simulink model "observer_tuning"  (R2016b)
settings: Solver=VariableStepAuto  StartTime=0.0  StopTime=10.0  RelTol=1e-3
values from neighbouring files (symbols this model uses):
  A = [0      1              0           0 ... (first row only)    [ImportStateSpace.m]    (also in multi_plot_tune_observer.m = sys.A; multi_plot_tune_observer2.m = sys.A; responseObserver.m = sys.A)
  B = [     0 ... (first row only)    [ImportStateSpace.m]    (also in multi_plot_tune_observer.m = sys.B; multi_plot_tune_observer2.m = sys.B; responseObserver.m = sys.B)
  C = [1 0 0 0 ... (first row only)    [ImportStateSpace.m]    (also in multi_plot_tune_observer.m = sys.C; multi_plot_tune_observer2.m = sys.C; responseObserver.m = sys.C)
  D = zeros(size(C,1), size(B,2))    [ImportStateSpace.m]    (also in multi_plot_tune_observer.m = sys.D; multi_plot_tune_observer2.m = sys.D; responseObserver.m = sys.D)
  K = place(sys.A, sys.B, eigs)    [LCSproject.m]    (also in myLQR.m = lqr(sys.A, sys.B, Q, R))
  kr = -1/(C*inv(A-B*K)*B)    [LCSproject.m]
  L_tuning = place(A',C',Poles)'    [multi_plot_tune_simulink_observer.m]
  simin_delay = 0.001    [multi_plot_tune_simulink_observer.m]
settings Model: Creator=Olivier  LastModifiedBy=Olivier

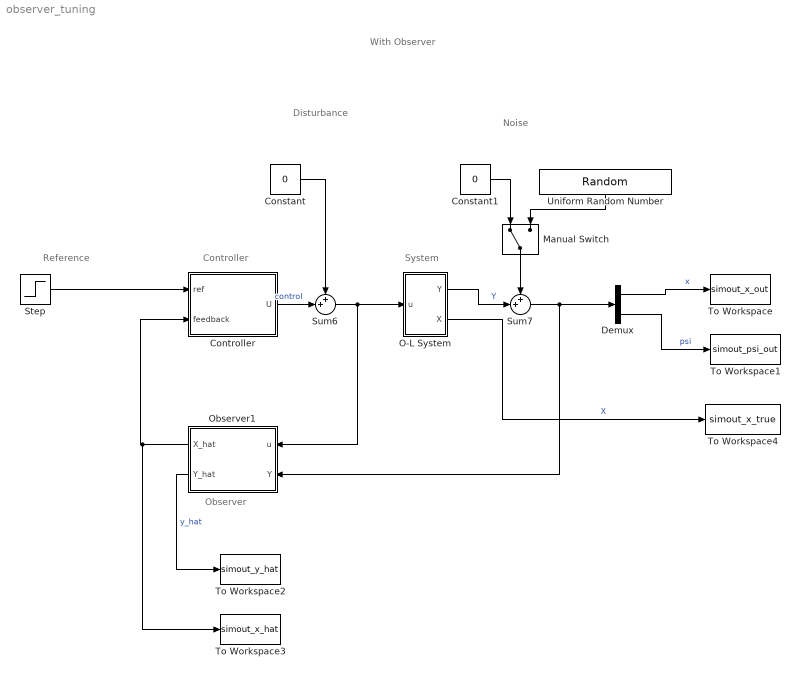
== system observer_tuning ==
  note: With Observer
  note: System
  note: Observer
  note: Controller
  note: Reference
  note: Disturbance
  note: Noise
  Constant : Constant  Value=0
  Constant1 : Constant  Value=0
  Controller : Subsystem
  Demux : Demux  Outputs=2
  Manual Switch : ManualSwitch
  O-L System : Subsystem
  Observer1 : Subsystem
  Step : Step  After=0.2  SampleTime=0
  Sum6 : Sum  Inputs=++|
  Sum7 : Sum  Inputs=++|
  To Workspace : ToWorkspace  VariableName=simout_x_out  SaveFormat=Timeseries  SampleTime=-1
  To Workspace1 : ToWorkspace  VariableName=simout_psi_out  SaveFormat=Timeseries  SampleTime=-1
  To Workspace2 : ToWorkspace  VariableName=simout_y_hat  SaveFormat=Timeseries  SampleTime=-1
  To Workspace3 : ToWorkspace  VariableName=simout_x_hat  SaveFormat=Timeseries  SampleTime=-1
  To Workspace4 : ToWorkspace  VariableName=simout_x_true  SaveFormat=Timeseries  SampleTime=-1
  Uniform Random Number : UniformRandomNumber  Minimum=-0.0001  Maximum=0.0001  SampleTime=0.1
  wires:
  Sum7/1 -> Demux/1, Observer1/2(Y)
  Controller/1(U) -> Sum6/2  "control"
  Observer1/1(X_hat) -> To Workspace3/1, Controller/2(feedback)
  Sum6/1 -> Observer1/1(u), O-L System/1(u)
  Manual Switch/1 -> Sum7/1
  Demux/2 -> To Workspace1/1  "psi"
  Demux/1 -> To Workspace/1  "x"
  O-L System/1(Y) -> Sum7/2  "Y"
  Step/1 -> Controller/1(ref)
  Observer1/2(Y_hat) -> To Workspace2/1  "y_hat"
  O-L System/2(X) -> To Workspace4/1  "X"
  Constant/1 -> Sum6/1
  Uniform Random Number/1 -> Manual Switch/2
  Constant1/1 -> Manual Switch/1

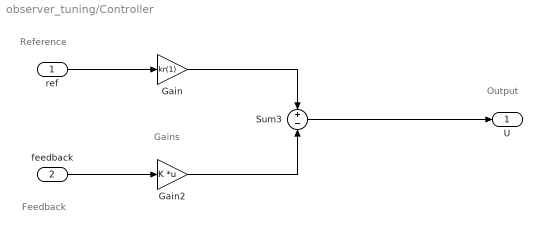
== system observer_tuning/Controller ==
  note: Output
  note: Gains
  note: Feedback
  note: Reference
  ref : Inport
  feedback : Inport  Port=2
  Gain : Gain  Gain=kr(1)
  Gain2 : Gain  Gain=K  Multiplication=Matrix(K*u)
  Sum3 : Sum  Inputs=+|-
  U : Outport
  wires:
  Sum3/1 -> U/1
  Gain2/1 -> Sum3/2
  feedback/1 -> Gain2/1
  ref/1 -> Gain/1
  Gain/1 -> Sum3/1

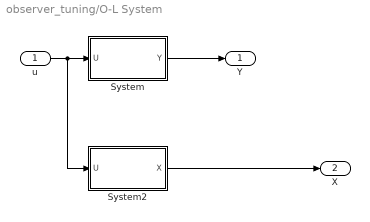
== system observer_tuning/O-L System ==
  u : Inport
  System : Subsystem
  System2 : Subsystem
  Y : Outport
  X : Outport  Port=2
  wires:
  System2/1(X) -> X/1
  System/1(Y) -> Y/1
  u/1 -> System2/1(U), System/1(U)

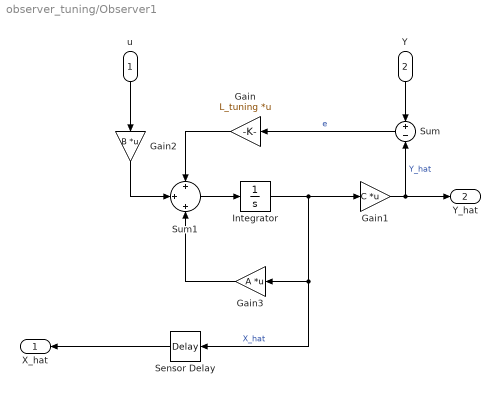
== system observer_tuning/Observer1 ==
  u : Inport
  Y : Inport  Port=2
  Gain : Gain  Gain=L_tuning  Multiplication=Matrix(K*u)
  Gain1 : Gain  Gain=C  Multiplication=Matrix(K*u)
  Gain2 : Gain  Gain=B  Multiplication=Matrix(K*u)
  Gain3 : Gain  Gain=A  Multiplication=Matrix(K*u)
  Integrator : Integrator
  Sensor Delay : TransportDelay  DelayTime=simin_delay
  Sum : Sum  Inputs=+|-
  Sum1 : Sum  Inputs=+|+|+
  X_hat : Outport
  Y_hat : Outport  Port=2
  wires:
  Sum/1 -> Gain/1  "e"
  Y/1 -> Sum/1
  Sum1/1 -> Integrator/1
  Integrator/1 -> Sensor Delay/1, Gain3/1, Gain1/1  "X_hat"
  Gain1/1 -> Y_hat/1, Sum/2  "Y_hat"
  Gain/1 -> Sum1/1
  u/1 -> Gain2/1
  Gain2/1 -> Sum1/2
  Gain3/1 -> Sum1/3
  Sensor Delay/1 -> X_hat/1

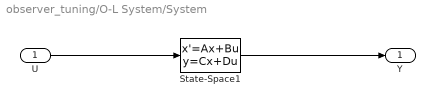
== system observer_tuning/O-L System/System ==
  U : Inport
  State-Space1 : StateSpace  A=A  B=B  C=C  D=D  X0=0
  Y : Outport
  wires:
  U/1 -> State-Space1/1
  State-Space1/1 -> Y/1

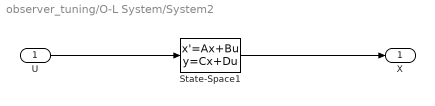
== system observer_tuning/O-L System/System2 ==
  U : Inport
  State-Space1 : StateSpace  A=A  B=B  C=eye(4)  D=[0;0;0;0]  X0=0
  X : Outport
  wires:
  U/1 -> State-Space1/1
  State-Space1/1 -> X/1
